simulink model "SimpleModel"  (R2021a)
settings: Solver=VariableStepAuto  StartTime=0.0  StopTime=10.0  RelTol=1e-3
undefined symbols (not defined in the file or in its folder): physconst, S
libraries: simrfV2util1 x3, simrfV2elements x2, simrfV2systems x1, simrfV2sources1 x1
settings Model: Creator=gzucchel  LastModifiedBy=gzucchel
settings DataIOCC: ExternalInput=externalInput_tp2ebfa4fc_d5b2_480b_ac9f_05a6fb0389d4  InitialState=initialState_tp2373128d_6ea1_457a_b053_e89f26a6a8c8  LoadExternalInput=on  SaveFinalState=on  SaveOperatingPoint=on  SaveFormat=Structure

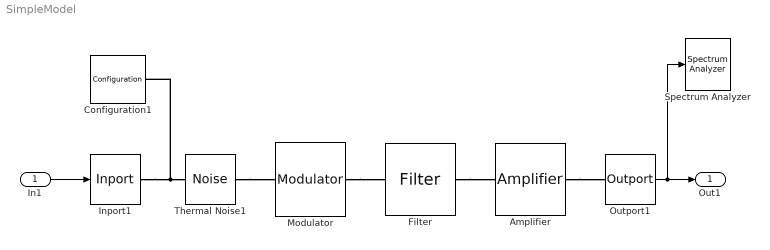
== system SimpleModel ==
  In1 : Inport  PortDimensions=1  SampleTime=1e-06  Interpolate=off
      settings: SignalType=complex
  Amplifier : simrfV2elements/Amplifier  classname=amplifier  DataSource=Data file  File=unitygain.s2p  Paramtype=S-parameters  Sparam=[0 0;1 0]  SparamFreq=1e9 Hz  SparamZ0=50  Residues=0  Poles=0  DF={0 0; 1 0}  Source_linear_gain=Available power gain  linear_gain=26 dB  Zin=50  Zout=50  Source_Poly=Even and odd order  Poly_Coeffs=[0 1]  IPType=Output  IP2=Inf dBm  IP3=10.1 dBm  P1dB=inf dBm  Psat=inf dBm  Gcomp=inf dBm  InternalGrounding=on  SourceFreq=Extracted from data source  PlotFreq=[1e9:1e6:3e9] Hz  PlotType=X-Y plane  YParam1=S(1,1)  YFormat1=Magnitude (decibels)  YParam2=None  YFormat2=Magnitude (decibels)  YOption=Linear  XOption=Linear  SparamRepresentation=Time domain (rationalfit)  FitTol=-40  FitOpt=Fit individually  AutoImpulseLength=on  ImpulseLength=1e-10 s  MagModeling=off  AddNoise=on  NoiseType=Noise figure  NoiseDist=White  NF=6  MinNF=0  Gopt=0  RN=0  CarrierFreq=0 Hz  NoiseAutoImpulseLength=on  NoiseImpulseLength=1e-10 s  SpecifyOpFreq=off  OpFreq=0 Hz
      settings: SourceProductBaseCode=RB
  Configuration1 : simrfV2util1/Configuration  AutoFreq=on  Tones=[] Hz  Harmonics=[]  NormalizeCarrierPower=on  SolverType=Auto  UseCCode=on  StepSize=1e-06 s  AddNoise=on  defaultRNG=on  Seed=0  Temperature=290.0 K  SolverDelFlag=0  AbsTol=1e-6  RelTol=1e-3  MaxIter=10  ErrorEstimationType=2-norm over all variables  EnableInterpFilter=on  HiddenFIRfilterControllerParam=on  SmallSignalApprox=off  AllSimFreqs=on  SimFreqs=[] Hz  SimFreqsInternal=[]  SamplesPerFrame=1
      settings: SourceProductBaseCode=RB
  Filter : simrfV2elements/Filter  classname=filter  DesignMethod=Butterworth  ResponseType=Bandpass  Implementation=LC Tee  ImplementationIdeal=Constant per carrier  ImplementationRational=Transfer function  UseFilterOrder=on  FilterOrder=3  PassFreq_lp=1 GHz  PassFreq_hp=2 GHz  PassFreq_bp=[2.04 2.16] GHz  PassFreq_bs=[1 4] GHz  PassAtten=3.0103  StopFreq_lp=2 GHz  StopFreq_hp=1 GHz  StopFreq_bp=[1.5 3.5] GHz  StopFreq_bs=[2.1 2.9] GHz  StopAtten=40  Rsrc=50  Rload=50  AutoImpulseLength=on  ImpulseLength=1e-10 s  InternalGrounding=on  PlotFuncLeft=Voltage transfer  PlotLeftForm=Magnitude (decibels)  PlotRightOnVT=None  PlotRightNoTD=None  PlotRightNoGD=None  PlotRightNoIR=None  PlotRightNoSR=None  PlotRightForm=Magnitude (decibels)  FreqPoints=logspace(0,10,101)  Freq_unit=Hz  TimePoints=linspace(0,1,1e6+1)  Time_unit=s  XaxisScale=Linear  YaxisScale=Linear  needRedraw=0
      settings: SourceProductBaseCode=RB
  Inport1 : simrfV2util1/Inport  SimulinkInputSignalType=Power  CarrierFreq=[100] MHz  ZS=50  InternalGrounding=on
      settings: SourceProductBaseCode=RB
  Modulator : simrfV2systems/Modulator  classname=rfmod  Source_linear_gain=Available power gain  linear_gain=-6 dB  Poly_Coeffs=[0 1]  LOFreq=2 GHz  Zin=50  Zout=50  AddIRFilter=on  AddCSFilter=on  InternalGrounding=on  ForceNextInit=off  Source_Poly=Even and odd order  IPType=Output  IP2=Inf dBm  IP3=12 dBm  P1dB=inf dBm  Psat=inf dBm  Gcomp=inf dBm  NF=2  Isolation=70 dB  AddPhaseNoise=on  PhaseNoiseOffset=[1e3 1e4 1e5 ]  PhaseNoiseLevel=[-80 -90 -120]  AutoImpulseLengthPN=on  ImpulseLengthPN=1e-10  ImpulseLength_unitPN=s  DesignMethodIR=Ideal  ResponseTypeIR=Lowpass  ImplementationIR=LC Tee  ImplementationIdealIR=Constant per carrier  ImplementationRationalIR=Transfer function  UseFilterOrderIR=on  FilterOrderIR=3  PassFreq_lpIR=150  PassFreq_lp_unitIR=MHz  PassFreq_hpIR=50  PassFreq_hp_unitIR=MHz  PassFreq_bpIR=[50 150]  PassFreq_bp_unitIR=MHz  PassFreq_bsIR=[4.049999999 4.150000001]  PassFreq_bs_unitIR=GHz  PassAttenIR=10*log10(2)  StopFreq_lpIR=150.000001  StopFreq_lp_unitIR=MHz  StopFreq_hpIR=49.999999  StopFreq_hp_unitIR=MHz  StopFreq_bpIR=[49.999999 150.000001]  StopFreq_bp_unitIR=MHz  StopFreq_bsIR=[4.05 4.15]  StopFreq_bs_unitIR=GHz  StopAttenIR=40  RsrcIR=50  RloadIR=50  AutoImpulseLengthIR=on  ImpulseLengthIR=1e-10  ImpulseLength_unitIR=s  DesignMethodCS=Ideal  ResponseTypeCS=Highpass  ImplementationCS=LC Tee  ImplementationIdealCS=Constant per carrier  ImplementationRationalCS=Transfer function  UseFilterOrderCS=on  FilterOrderCS=3  PassFreq_lpCS=2.15  PassFreq_lp_unitCS=GHz  PassFreq_hpCS=2.05  PassFreq_hp_unitCS=GHz  PassFreq_bpCS=[2.05 2.15]  PassFreq_bp_unitCS=GHz  PassFreq_bsCS=[1.849999999 1.950000001]  PassFreq_bs_unitCS=GHz  PassAttenCS=10*log10(2)  StopFreq_lpCS=2.150000001  StopFreq_lp_unitCS=GHz  StopFreq_hpCS=2.049999999  StopFreq_hp_unitCS=GHz  StopFreq_bpCS=[2.049999999 2.150000001]  StopFreq_bp_unitCS=GHz  StopFreq_bsCS=[1.85 1.95]  StopFreq_bs_unitCS=GHz  StopAttenCS=40  RsrcCS=50  RloadCS=50  AutoImpulseLengthCS=on  ImpulseLengthCS=1e-10  ImpulseLength_unitCS=s
      settings: SourceProductBaseCode=RB
  Outport1 : simrfV2util1/Outport  SensorType=Power  OutputFormat=Complex Baseband  CarrierFreq=[2.1] GHz  ZL=50  InternalGrounding=on  StepSize=1e-6 s  AutoStep=on
      settings: SourceProductBaseCode=RB
  Spectrum Analyzer : SpectrumAnalyzer
  Thermal Noise1 : simrfV2sources1/Noise  SimulinkInputSignalType=Ideal voltage  NoiseType=White  NoisePSD=4*physconst('Boltzmann')*290*50  CarrierFreq=0 Hz  AutoImpulseLength=on  ImpulseLength=1e-10 s  InternalGrounding=off
      settings: SourceProductBaseCode=RB
  Out1 : Outport  PortDimensions=1  SampleTime=1e-06
  wires:
  In1/1 -> Inport1/1
  Outport1/1 -> Spectrum Analyzer/1, Out1/1
  connections:
  Configuration1/LConn1 -- Inport1/RConn1 -- Thermal Noise1/RConn1
  Thermal Noise1/LConn1 -- Modulator/LConn1
  Modulator/RConn1 -- Filter/LConn1
  Filter/RConn1 -- Amplifier/LConn1
  Amplifier/RConn1 -- Outport1/LConn1
